simulink model "FullStateFeedBack"  (R2016b)
settings: Solver=VariableStepAuto  StartTime=0.0  StopTime=10.0  RelTol=1e-3
values from neighbouring files (symbols this model uses):
  A = [0      1              0           0 ... (first row only)    [InitFile.m]
  B = [     0 ... (first row only)    [InitFile.m]
  C = [1 0 0 0 ... (first row only)    [InitFile.m]
  D = [0 ... (first row only)    [InitFile.m]
undefined symbols (not defined in the file or in its folder): Ke, x0
settings Model: Creator=AHKh  LastModifiedBy=AHKh

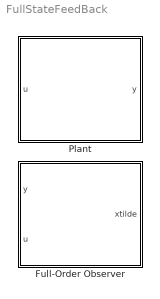
== system FullStateFeedBack ==
  Full-Order Observer : Subsystem  mask{x0=x0, A=A, B=B, C=C, D=D}
      mask prompts: x0 "Initial States"; A "System Matrix (A)"; B "Input Matrix (B)"; C "State-Output Matrix (C)"; D "Input-Output Matrix (D)"
  Plant : Subsystem  mask{x0=x0, A=A, B=B, C=C, D=D}
      mask prompts: x0 "Initial States"; A "System Matrix (A)"; B "Input Matrix (B)"; C "State-Output Matrix (C)"; D "Input-Output Matrix (D)"

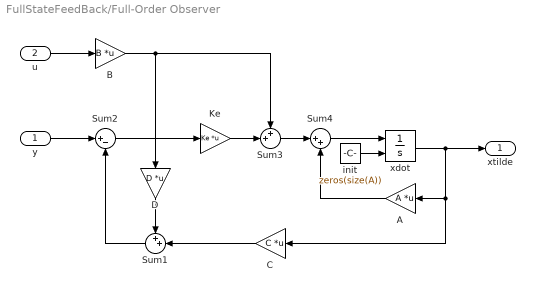
== system FullStateFeedBack/Full-Order Observer ==
  y : Inport
  u : Inport  Port=2
  A : Gain  Gain=A  Multiplication=Matrix(K*u)
  B : Gain  Gain=B  Multiplication=Matrix(K*u)
  C : Gain  Gain=C  Multiplication=Matrix(K*u)
  D : Gain  Gain=D  Multiplication=Matrix(K*u)
  Ke : Gain  Gain=Ke  Multiplication=Matrix(K*u)
  Sum1 : Sum  Inputs=++|
  Sum2 : Sum  Inputs=|+-
  Sum3 : Sum  Inputs=++|
  Sum4 : Sum  Inputs=|++
  init : Constant  Value=zeros(size(A))
  xdot : Integrator  InitialConditionSource=external
  xtilde : Outport
  wires:
  y/1 -> Sum2/1
  u/1 -> B/1
  Sum2/1 -> Ke/1
  Ke/1 -> Sum3/2
  B/1 -> Sum3/1, D/1
  init/1 -> xdot/2
  xdot/1 -> xtilde/1, A/1, C/1
  Sum4/1 -> xdot/1
  A/1 -> Sum4/2
  Sum3/1 -> Sum4/1
  C/1 -> Sum1/2
  D/1 -> Sum1/1
  Sum1/1 -> Sum2/2

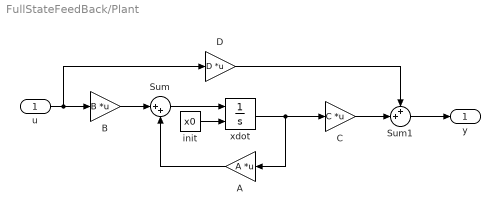
== system FullStateFeedBack/Plant ==
  u : Inport
  A : Gain  Gain=A  Multiplication=Matrix(K*u)
  B : Gain  Gain=B  Multiplication=Matrix(K*u)
  C : Gain  Gain=C  Multiplication=Matrix(K*u)
  D : Gain  Gain=D  Multiplication=Matrix(K*u)
  Sum : Sum  Inputs=|++
  Sum1 : Sum  Inputs=++|
  init : Constant  Value=x0
  xdot : Integrator  InitialConditionSource=external
  y : Outport
  wires:
  u/1 -> D/1, B/1
  B/1 -> Sum/1
  A/1 -> Sum/2
  Sum/1 -> xdot/1
  xdot/1 -> C/1, A/1
  init/1 -> xdot/2
  C/1 -> Sum1/2
  Sum1/1 -> y/1
  D/1 -> Sum1/1
